simulink model "siddhant_suspension_modelling"  (R2014a)
settings: Solver=ode45  StartTime=0.0  StopTime=50  RelTol=1e-3
settings Model: Creator=user  LastModifiedBy=user

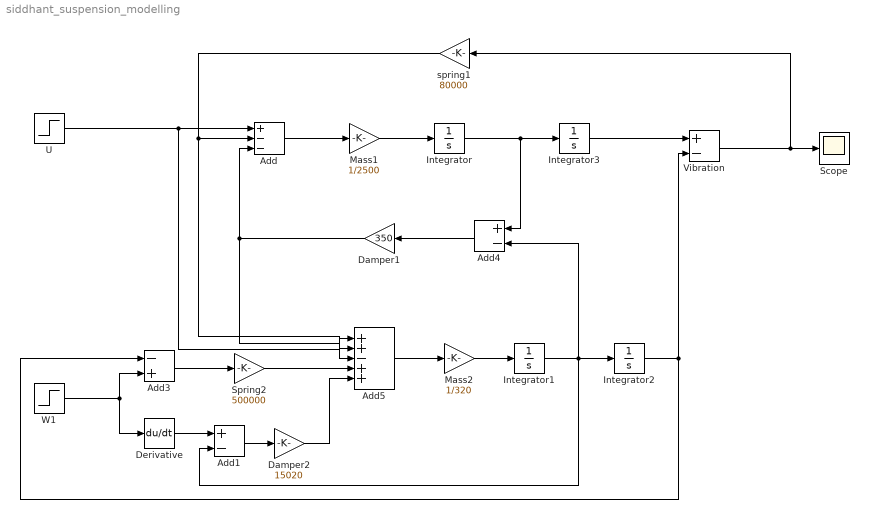
== system siddhant_suspension_modelling ==
  Add : Sum  Inputs=+--
  Add1 : Sum  Inputs=+-
  Add3 : Sum  Inputs=-+
  Add4 : Sum  Inputs=+-
  Add5 : Sum  Inputs=++-++  RndMeth=Nearest
  "Damper1 " : Gain  Gain=350
  Damper2 : Gain  Gain=15020
  Derivative : Derivative
  Integrator{,1..3} (4 alike) : Integrator
  Mass1 : Gain  Gain=1/2500
  Mass2 : Gain  Gain=1/320
  Scope : Scope
      settings: ShowLegends=on
  Spring2 : Gain  Gain=500000
  U : Step  Time=0  SampleTime=0
  "Vibration " : Sum  Inputs=+-
  W1 : Step  Time=0  SampleTime=0
  spring1 : Gain  Gain=80000
  wires:
  U/1 -> Add5/3, Add/1
  Add/1 -> Mass1/1
  Mass1/1 -> Integrator/1
  Integrator/1 -> Add4/1, Integrator3/1
  Integrator3/1 -> "Vibration "/1
  "Vibration "/1 -> spring1/1, Scope/1
  W1/1 -> Add3/2, Derivative/1
  Integrator2/1 -> Add3/1, "Vibration "/2
  Add4/1 -> "Damper1 "/1
  Add3/1 -> Spring2/1
  Spring2/1 -> Add5/4
  Add5/1 -> Mass2/1
  Mass2/1 -> Integrator1/1
  Integrator1/1 -> Add1/2, Add4/2, Integrator2/1
  Damper2/1 -> Add5/5
  Add1/1 -> Damper2/1
  Derivative/1 -> Add1/1
  "Damper1 "/1 -> Add/3, Add5/1
  spring1/1 -> Add/2, Add5/2
